simulink model "voltage_controller"  (R2022a)
settings: Solver=FixedStepAuto  StartTime=0.0  StopTime=1  FixedStep=3e-8  RelTol=1e-3
values from neighbouring files (symbols this model uses):
  fs = 50*10^3    (= 50000)    [current_controller_parameters.m]
  I_gain_voltage = 1.8226e-4    (= 0.00018226)    [current_controller_parameters.m]
  Kii = 0.0307    [current_controller_parameters.m]
  Kpi = 9.65    [current_controller_parameters.m]
  P_gain_voltage = 0.148    [current_controller_parameters.m]
libraries: spsCurrentMeasurementLib x7, simulink x4, spsMosfetLib x4, spsSeriesRLCBranchLib x4, spsVoltageMeasurementLib x3, spsACVoltageSourceLib x1, spspowerguiLib x1
settings Model: Creator=RTX  LastModifiedBy=RTX

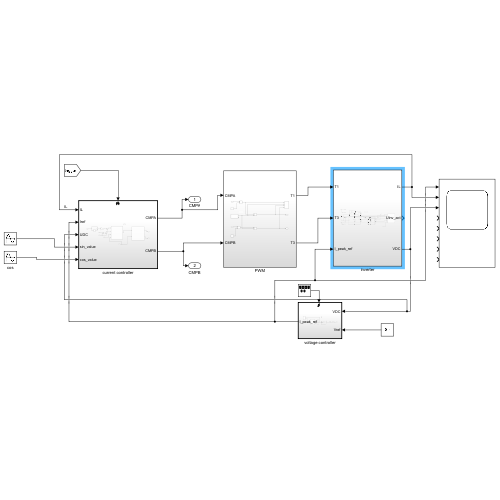
[thumbnail: Simulink's stored preview of the top-level diagram]
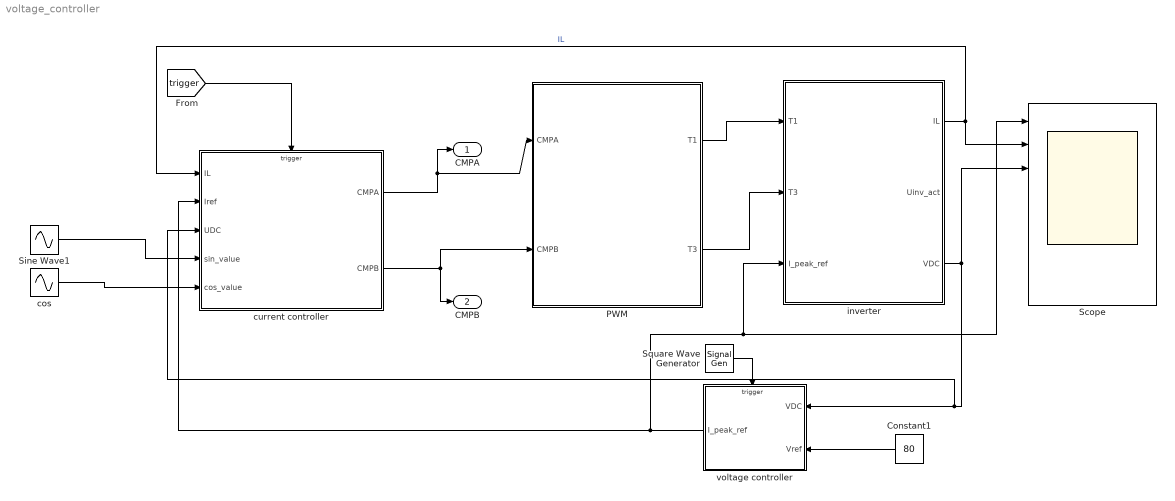
== system voltage_controller ==
  Constant1 : Constant  Value=80
  PWM : Subsystem
  Scope : Scope  NumInputPorts=8
  Sine Wave1 : Sin  Frequency=2*pi*50  Phase=-0.03778  SampleTime=0
  Square Wave Generator : SignalGenerator  WaveForm=square  Frequency=10000
  cos : Sin  Frequency=2*pi*50  Phase=pi/2-0.03778  SampleTime=0
  current controller : Subsystem
  inverter : Subsystem
  voltage controller : Subsystem
  CMPA : Outport
  CMPB : Outport  Port=2
  wires:
  inverter/3(VDC) -> Scope/3, voltage controller/1(VDC), current controller/3(UDC)
  [trigger] -> current controller/Trigger
  current controller/2(CMPB) -> PWM/2(CMPB), CMPB/1
  cos/1 -> current controller/5(cos_value)
  PWM/1(T1) -> inverter/1(T1)
  current controller/1(CMPA) -> CMPA/1, PWM/1(CMPA)
  PWM/2(T3) -> inverter/2(T3)
  Sine Wave1/1 -> current controller/4(sin_value)
  inverter/1(IL) -> current controller/1(IL), Scope/2  "IL"
  voltage controller/1(I_peak_ref) -> Scope/1, inverter/3(I_peak_ref), current controller/2(Iref)
  Constant1/1 -> voltage controller/2(Vref)
  Square Wave Generator/1 -> voltage controller/Trigger

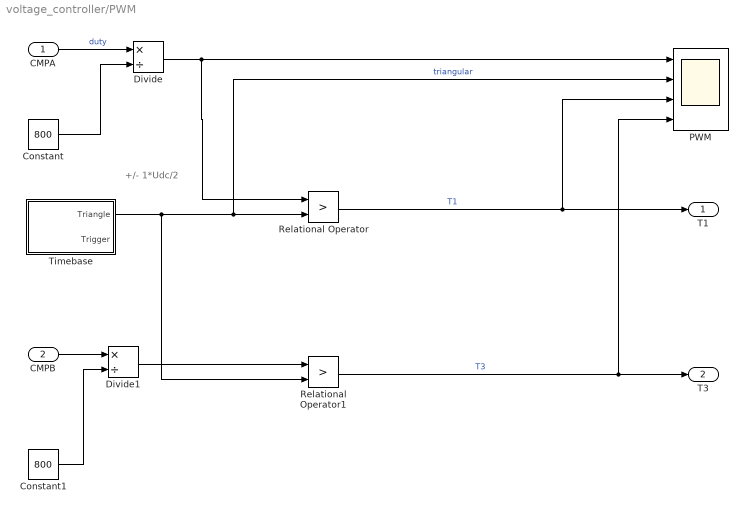
== system voltage_controller/PWM ==
  note: +/- 1*Udc/2
  CMPA : Inport
  CMPB : Inport  Port=2
  Constant : Constant  Value=800
  Constant1 : Constant  Value=800
  Divide : Product  Inputs=*/
  Divide1 : Product  Inputs=*/
  PWM : Scope  NumInputPorts=4
  Relational Operator : RelationalOperator  Operator=>  OutDataTypeStr=boolean  InputSameDT=off
  Relational Operator1 : RelationalOperator  Operator=>  OutDataTypeStr=boolean  InputSameDT=off
  Timebase : Subsystem
  T1 : Outport
  T3 : Outport  Port=2
  wires:
  Timebase/1(Triangle) -> Relational Operator1/2, Relational Operator/2, PWM/2  "triangular"
  Relational Operator/1 -> T1/1, PWM/3  "T1"
  Relational Operator1/1 -> T3/1, PWM/4  "T3"
  Constant/1 -> Divide/2
  Divide/1 -> Relational Operator/1, PWM/1
  CMPA/1 -> Divide/1  "duty"
  CMPB/1 -> Divide1/1
  Constant1/1 -> Divide1/2
  Divide1/1 -> Relational Operator1/1

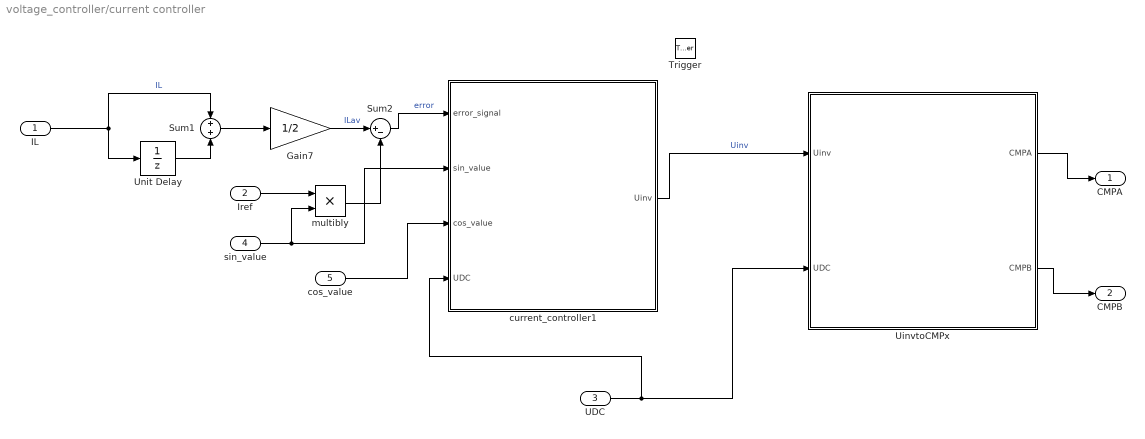
== system voltage_controller/current controller ==
  IL : Inport
  Iref : Inport  Port=2
  UDC : Inport  Port=3
  sin_value : Inport  Port=4
  cos_value : Inport  Port=5
  Trigger : TriggerPort  TriggerType=either  VariantControl=(inherit)
  Gain7 : Gain  Gain=1/2
  Sum1 : Sum  Inputs=+|+
  Sum2 : Sum  Inputs=|+-
  UinvtoCMPx : Subsystem
  Unit Delay : UnitDelay  SampleTime=-1  HasFrameUpgradeWarning=on
  current_controller1 : Subsystem
  multibly : Product  Inputs=**
  CMPA : Outport
  CMPB : Outport  Port=2
  wires:
  current_controller1/1(Uinv) -> UinvtoCMPx/1(Uinv)  "Uinv"
  cos_value/1 -> current_controller1/3(cos_value)
  sin_value/1 -> current_controller1/2(sin_value), multibly/2
  UinvtoCMPx/1(CMPA) -> CMPA/1
  UinvtoCMPx/2(CMPB) -> CMPB/1
  Unit Delay/1 -> Sum1/2
  IL/1 -> Sum1/1, Unit Delay/1  "IL"
  Sum1/1 -> Gain7/1
  Gain7/1 -> Sum2/1  "ILav"
  multibly/1 -> Sum2/2
  Sum2/1 -> current_controller1/1(error_signal)  "error"
  Iref/1 -> multibly/1
  UDC/1 -> current_controller1/4(UDC), UinvtoCMPx/2(UDC)

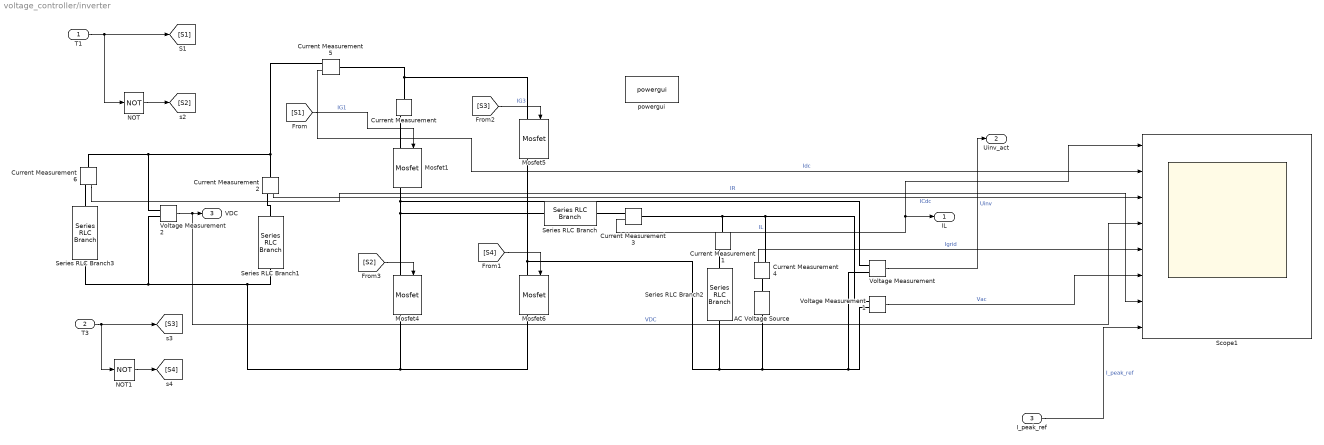
== system voltage_controller/inverter ==
  T1 : Inport
  T3 : Inport  Port=2
  I_peak_ref : Inport  Port=3
  AC Voltage Source : spsACVoltageSourceLib/AC Voltage Source  Amplitude=40*sqrt(2)  Phase=0  Frequency=50  SampleTime=0  Measurements=None  BusType=swing  Pref=10e3  Qref=0  Qmin=-inf  Qmax=+inf
  Current Measurement{,1..6} (7 alike) : spsCurrentMeasurementLib/Current Measurement  PhasorSimulation=off  OutputType=Complex  PSBequivalent=0
  Mosfet{1,4..6} (4 alike) : spsMosfetLib/Mosfet  Ron=.1  Lon=0  Rd=.01  Vfd=0  IC=0  Rs=1e5  Cs=inf  Measurements=on
  NOT : Logic  Operator=NOT  IconShape=distinctive  AllPortsSameDT=off  OutDataTypeStr=boolean
  NOT1 : Logic  Operator=NOT  IconShape=distinctive  AllPortsSameDT=off  OutDataTypeStr=boolean
  Scope1 : Scope  NumInputPorts=8
  Series RLC Branch : spsSeriesRLCBranchLib/Series RLC Branch  LConnTagsString=__new0  RConnTagsString=__new0  BranchType=RL  Resistance=0.001  Inductance=600*10^-6  SetiL0=off  InitialCurrent=0  Capacitance=1e-6  Setx0=off  InitialVoltage=0  Measurements=None
  Series RLC Branch1 : spsSeriesRLCBranchLib/Series RLC Branch  LConnTagsString=__new0  RConnTagsString=__new0  BranchType=RC  Resistance=0.001  Inductance=4.06e-3  SetiL0=off  InitialCurrent=0  Capacitance=800e-6  Setx0=on  InitialVoltage=48*sqrt(2)  Measurements=None
  Series RLC Branch2 : spsSeriesRLCBranchLib/Series RLC Branch  LConnTagsString=__new0  RConnTagsString=__new0  BranchType=RC  Resistance=0.001  Inductance=4.06e-3  SetiL0=off  InitialCurrent=0  Capacitance=16e-6  Setx0=on  InitialVoltage=0  Measurements=None
  Series RLC Branch3 : spsSeriesRLCBranchLib/Series RLC Branch  LConnTagsString=__new0  RConnTagsString=__new0  BranchType=R  Resistance=60  Inductance=4.06e-3  SetiL0=off  InitialCurrent=0  Capacitance=800e-6  Setx0=on  InitialVoltage=90  Measurements=None
  Voltage Measurement : spsVoltageMeasurementLib/Voltage Measurement  PhasorSimulation=off  OutputType=Complex  PSBequivalent=0
  Voltage Measurement1 : spsVoltageMeasurementLib/Voltage Measurement  PhasorSimulation=off  OutputType=Complex  PSBequivalent=0
  Voltage Measurement2 : spsVoltageMeasurementLib/Voltage Measurement  PhasorSimulation=off  OutputType=Complex  PSBequivalent=0
  powergui : spspowerguiLib/powergui  Priority=1  SimulationMode=Continuous  SampleTime=50e-6  frequency=60  Iterations=50  frequencyindice=50  Pbase=100e6  ErrMax=1e-4  UnitsV=kV  UnitsW=MW  buscounter=0  FunctionMessages=off  echomessages=off  EnableUseOfTLC=off  CurrentSourceSwitches=off  DisableSnubberDevices=off  DisableRonSwitches=off  DisableVfSwitches=off  DisplayEquations=off  AutomaticDiscreteSolvers=off  SolverType=Tustin/Backward Euler (TBE)  Interpol=off  ExternalGateDelay=off  methode=off  Ts=100  x0status=blocks  SPID=on  SwTol=0  HookPort=off  NonlinearTolerance=1e-4  nMaxIteration=100  ContinueOnMaxIteration=off  RestoreLinks=warning  ResistiveCurrentMeasurement=off  Frange=[0:2:500]  Ylog=off  Xlog=on  ShowGrid=off  save=off  variable=ZData  structure=0  ZoomFFT=off  StartTime=0.0  cycles=1  DisplayStyle=1  fundamental=60  FreqAxis=off  MaxFrequency=1000  frequencyindicesteady=1  RmsSteady=1  display=off
  IL : Outport
  Uinv_act : Outport  Port=2
  VDC : Outport  Port=3
  wires:
  Current Measurement3/1 -> Scope1/1, IL/1  "IL"
  Current Measurement2/1 -> Scope1/3  "ICdc"
  [S4] -> Mosfet6/1
  Voltage Measurement/1 -> Uinv_act/1  "Uinv"
  [S2] -> Mosfet4/1
  [S3] -> Mosfet5/1  "IG3"
  [S1] -> Mosfet1/1  "IG1"
  T3/1 -> [S3], NOT1/1
  T1/1 -> [S1], NOT/1
  NOT1/1 -> [S4]
  NOT/1 -> [S2]
  Voltage Measurement1/1 -> Scope1/6  "Vac"
  Voltage Measurement2/1 -> Scope1/4, VDC/1  "VDC"
  Current Measurement4/1 -> Scope1/5  "Igrid"
  Current Measurement5/1 -> Scope1/2  "Idc"
  Current Measurement6/1 -> Scope1/7  "IR"
  I_peak_ref/1 -> Scope1/8  "I_peak_ref"
  connections:
  Current Measurement1/LConn1 -- Voltage Measurement1/LConn1 -- Current Measurement4/RConn1 -- Current Measurement3/LConn1
  Series RLC Branch1/RConn1 -- Mosfet6/RConn1 -- Mosfet4/RConn1 -- Series RLC Branch3/RConn1 -- Voltage Measurement2/LConn2
  Current Measurement/LConn1 -- Current Measurement5/LConn1 -- Mosfet5/LConn1
  Voltage Measurement/LConn1 -- Mosfet4/LConn1 -- Series RLC Branch/LConn1 -- Mosfet1/RConn1
  Voltage Measurement2/LConn1 -- Current Measurement5/RConn1 -- Current Measurement2/LConn1 -- Current Measurement6/LConn1
  Mosfet1/LConn1 -- Current Measurement/RConn1
  Current Measurement1/RConn1 -- Series RLC Branch2/LConn1
  Series RLC Branch/RConn1 -- Current Measurement3/RConn1
  Series RLC Branch2/RConn1 -- AC Voltage Source/LConn1 -- Voltage Measurement1/LConn2 -- Voltage Measurement/LConn2 -- Mosfet6/LConn1 -- Mosfet5/RConn1
  AC Voltage Source/RConn1 -- Current Measurement4/LConn1
  Series RLC Branch3/LConn1 -- Current Measurement6/RConn1
  Series RLC Branch1/LConn1 -- Current Measurement2/RConn1

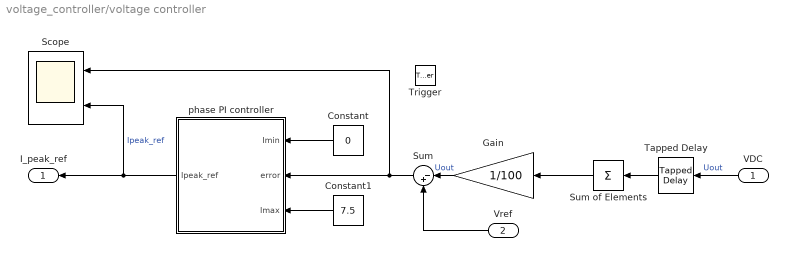
== system voltage_controller/voltage controller ==
  VDC : Inport
  Vref : Inport  Port=2
  Trigger : TriggerPort  VariantControl=(inherit)  PortDimensions=1
  Constant : Constant  Value=0
  Constant1 : Constant  Value=7.5
  Gain : Gain  Gain=1/100
  Scope : Scope  NumInputPorts=2
  Sum : Sum  Inputs=|-+
  Sum of Elements : Sum  Inputs=+
  Tapped Delay : simulink/Discrete/Tapped Delay  vinit=26  samptime=-1  NumDelays=100  DelayOrder=Oldest  includeCurrent=off
  phase PI controller : Subsystem
  I_peak_ref : Outport
  wires:
  Vref/1 -> Sum/2
  Sum/1 -> Scope/1, phase PI controller/2(error)
  Constant/1 -> phase PI controller/1(Imin)
  Constant1/1 -> phase PI controller/3(Imax)
  phase PI controller/1(Ipeak_ref) -> Scope/2, I_peak_ref/1  "Ipeak_ref"
  Sum of Elements/1 -> Gain/1
  Tapped Delay/1 -> Sum of Elements/1
  VDC/1 -> Tapped Delay/1  "Uout"
  Gain/1 -> Sum/1  "Uout"

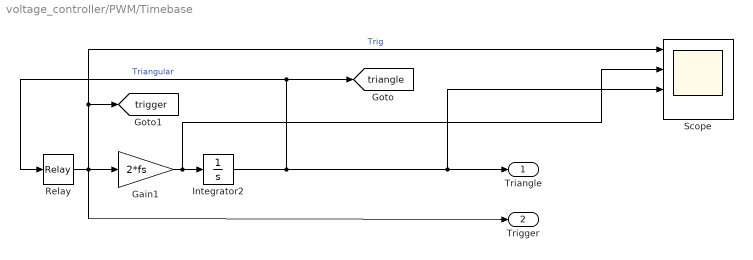
== system voltage_controller/PWM/Timebase ==
  Gain1 : Gain  Gain=2*fs
  Integrator2 : Integrator  LowerSaturationLimit=0
  Relay : Relay  OnSwitchValue=1  OffSwitchValue=0  OnOutputValue=-1  OffOutputValue=1
  Scope : Scope  NumInputPorts=4
  Triangle : Outport  VectorParamsAs1DForOutWhenUnconnected=off
  Trigger : Outport  Port=2  VectorParamsAs1DForOutWhenUnconnected=off
  tag scope: triangle=global, trigger=global
  wires:
  Integrator2/1 -> Scope/3, Triangle/1, [triangle], Relay/1  "Triangular"
  Relay/1 -> Gain1/1, [trigger], Scope/1, Trigger/1  "Trig"
  Gain1/1 -> Scope/2, Integrator2/1

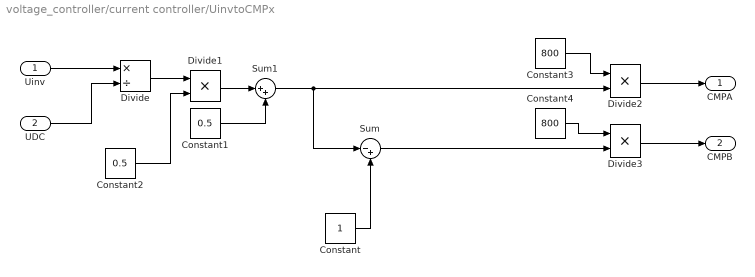
== system voltage_controller/current controller/UinvtoCMPx ==
  Uinv : Inport
  UDC : Inport  Port=2
  Constant : Constant
  Constant1 : Constant  Value=0.5
  Constant2 : Constant  Value=0.5
  Constant3 : Constant  Value=800
  Constant4 : Constant  Value=800
  Divide : Product  Inputs=*/
  Divide1 : Product  Inputs=**
  Divide2 : Product  Inputs=**
  Divide3 : Product  Inputs=**
  Sum : Sum  Inputs=|-+
  Sum1 : Sum  Inputs=|++
  CMPA : Outport
  CMPB : Outport  Port=2
  wires:
  Divide2/1 -> CMPA/1
  Sum/1 -> Divide3/2
  Constant/1 -> Sum/2
  Uinv/1 -> Divide/1
  UDC/1 -> Divide/2
  Divide/1 -> Divide1/1
  Constant2/1 -> Divide1/2
  Divide1/1 -> Sum1/1
  Constant1/1 -> Sum1/2
  Sum1/1 -> Sum/1, Divide2/2
  Constant3/1 -> Divide2/1
  Constant4/1 -> Divide3/1
  Divide3/1 -> CMPB/1

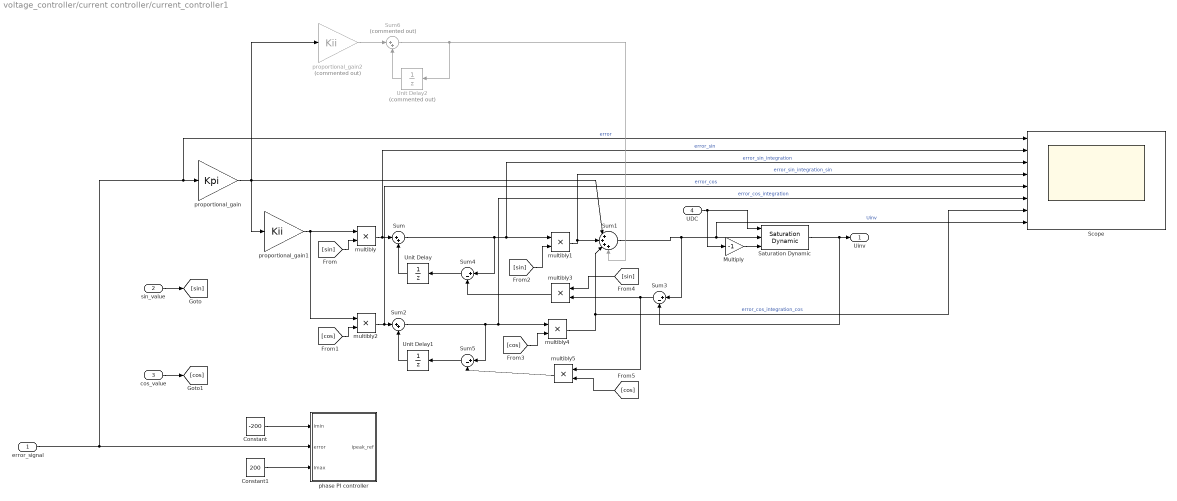
== system voltage_controller/current controller/current_controller1 ==
  error_signal : Inport
  sin_value : Inport  Port=2
  cos_value : Inport  Port=3
  UDC : Inport  Port=4
  Constant : Constant  Value=-200
  Constant1 : Constant  Value=200
  Multiply : Gain  Gain=-1
  Saturation Dynamic : simulink/Discontinuities/Saturation Dynamic  OutMin=[]  OutMax=[]  OutDataTypeStr=Inherit: Same as second input  OutDataType=fixdt(1, 16)  OutScaling=2^-10  DoSatur=off
  Scope : Scope  NumInputPorts=8
  Sum : Sum  Inputs=|++
  Sum1 : Sum  Inputs=|++++
  Sum2 : Sum  Inputs=|++
  Sum3 : Sum  Inputs=|+-
  Sum4 : Sum  Inputs=|+-
  Sum5 : Sum  Inputs=|+-
  Sum6 : Sum  Commented=on  Inputs=|++
  Unit Delay : UnitDelay  InitialCondition=48*sqrt(2)  SampleTime=-1  HasFrameUpgradeWarning=on
  Unit Delay1 : UnitDelay  SampleTime=-1  HasFrameUpgradeWarning=on
  Unit Delay2 : UnitDelay  Commented=on  SampleTime=-1  HasFrameUpgradeWarning=on
  multibly{,1..5} (6 alike) : Product  Inputs=**
  phase PI controller : Subsystem
  proportional_gain : Gain  Gain=Kpi
  proportional_gain1 : Gain  Gain=Kii
  proportional_gain2 : Gain  Commented=on  Gain=Kii
  Uinv : Outport
  wires:
  proportional_gain/1 -> proportional_gain2/1, Sum1/1, proportional_gain1/1
  Saturation Dynamic/1 -> Sum3/2, Uinv/1
  error_signal/1 -> phase PI controller/2(error), Scope/1, proportional_gain/1  "error"
  Sum2/1 -> Sum5/1, Scope/6, multibly4/1  "error_cos_integration"
  [cos] -> multibly4/2
  multibly5/1 -> Sum5/2
  [cos] -> multibly2/2
  multibly/1 -> Scope/2, Sum/1  "error_sin"
  Unit Delay/1 -> Sum/2
  Sum4/1 -> Unit Delay/1
  multibly4/1 -> Scope/7, Sum1/3  "error_cos_integration_cos"
  [sin] -> multibly/2
  Sum3/1 -> multibly5/1, multibly3/2
  Unit Delay1/1 -> Sum2/2
  Sum/1 -> Sum4/1, Scope/3, multibly1/1  "error_sin_integration"
  sin_value/1 -> [sin]
  proportional_gain1/1 -> multibly2/1, multibly/1
  Sum1/1 -> Scope/8, Saturation Dynamic/2, Sum3/1  "Uinv"
  multibly2/1 -> Scope/5, Sum2/1  "error_cos"
  Sum5/1 -> Unit Delay1/1
  multibly3/1 -> Sum4/2
  [cos] -> multibly5/2
  [sin] -> multibly3/1
  cos_value/1 -> [cos]
  [sin] -> multibly1/2
  multibly1/1 -> Scope/4, Sum1/2  "error_sin_integration_sin"
  Constant1/1 -> phase PI controller/3(Imax)
  Constant/1 -> phase PI controller/1(Imin)
  proportional_gain2/1 -> Sum6/1
  Sum6/1 -> Sum1/4, Unit Delay2/1
  Unit Delay2/1 -> Sum6/2
  UDC/1 -> Saturation Dynamic/1, Multiply/1
  Multiply/1 -> Saturation Dynamic/3

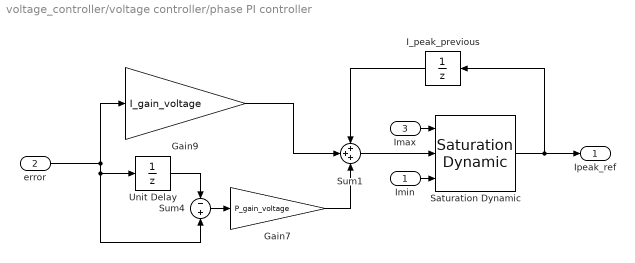
== system voltage_controller/voltage controller/phase PI controller ==
  Imin : Inport
  error : Inport  Port=2
  Imax : Inport  Port=3
  Gain7 : Gain  Gain=P_gain_voltage
  Gain9 : Gain  Gain=I_gain_voltage
  I_peak_previous : UnitDelay  SampleTime=-1  HasFrameUpgradeWarning=on
  Saturation Dynamic : simulink/Discontinuities/Saturation Dynamic  OutMin=[]  OutMax=[]  OutDataTypeStr=Inherit: Same as second input  OutDataType=fixdt(1, 16)  OutScaling=2^-10  DoSatur=off
  Sum1 : Sum  Inputs=+++
  Sum4 : Sum  Inputs=-|+
  Unit Delay : UnitDelay  SampleTime=-1  HasFrameUpgradeWarning=on
  Ipeak_ref : Outport  VectorParamsAs1DForOutWhenUnconnected=off
  wires:
  I_peak_previous/1 -> Sum1/1
  Gain9/1 -> Sum1/2
  Imax/1 -> Saturation Dynamic/1
  Sum1/1 -> Saturation Dynamic/2
  Saturation Dynamic/1 -> Ipeak_ref/1, I_peak_previous/1
  Imin/1 -> Saturation Dynamic/3
  Unit Delay/1 -> Sum4/1
  error/1 -> Gain9/1, Unit Delay/1, Sum4/2
  Sum4/1 -> Gain7/1
  Gain7/1 -> Sum1/3

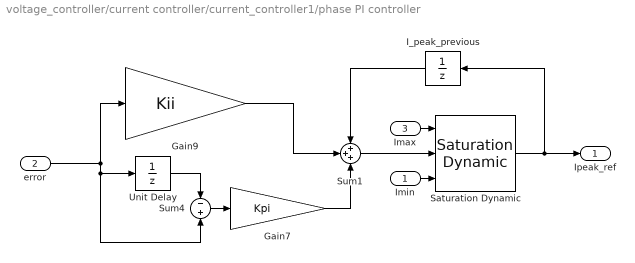
== system voltage_controller/current controller/current_controller1/phase PI controller ==
  Imin : Inport
  error : Inport  Port=2
  Imax : Inport  Port=3
  Gain7 : Gain  Gain=Kpi
  Gain9 : Gain  Gain=Kii
  I_peak_previous : UnitDelay  SampleTime=-1  HasFrameUpgradeWarning=on
  Saturation Dynamic : simulink/Discontinuities/Saturation Dynamic  OutMin=[]  OutMax=[]  OutDataTypeStr=Inherit: Same as second input  OutDataType=fixdt(1, 16)  OutScaling=2^-10  DoSatur=off
  Sum1 : Sum  Inputs=+++
  Sum4 : Sum  Inputs=-|+
  Unit Delay : UnitDelay  SampleTime=-1  HasFrameUpgradeWarning=on
  Ipeak_ref : Outport  VectorParamsAs1DForOutWhenUnconnected=off
  wires:
  I_peak_previous/1 -> Sum1/1
  Gain9/1 -> Sum1/2
  Imax/1 -> Saturation Dynamic/1
  Sum1/1 -> Saturation Dynamic/2
  Saturation Dynamic/1 -> Ipeak_ref/1, I_peak_previous/1
  Imin/1 -> Saturation Dynamic/3
  Unit Delay/1 -> Sum4/1
  error/1 -> Gain9/1, Unit Delay/1, Sum4/2
  Sum4/1 -> Gain7/1
  Gain7/1 -> Sum1/3
